simulink model "lab5_ss_decoupler"  (R2022b)
settings: Solver=VariableStepAuto  StartTime=0.0  StopTime=10.0  RelTol=1e-3
settings Model: Creator=qm-zhu  LastModifiedBy=ASUS
settings SolverCC: AlgebraicLoopSolver=TrustRegion
settings DebuggingCC: UnconnectedInputMsg=warning  UnconnectedOutputMsg=warning  UnconnectedLineMsg=warning  SFMachineParentedDataDiag=warning
settings ModelReferenceCC: EnableRefExpFcnMdlSchedulingChecks=on
settings SFSimCC: CustomCodeUndefinedFunction=UseInterfaceOnly

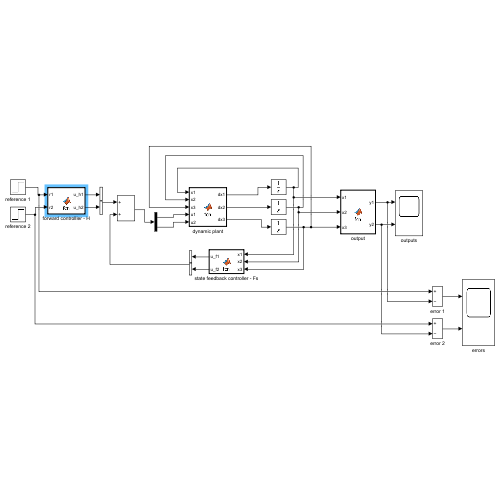
[thumbnail: Simulink's stored preview of the top-level diagram]
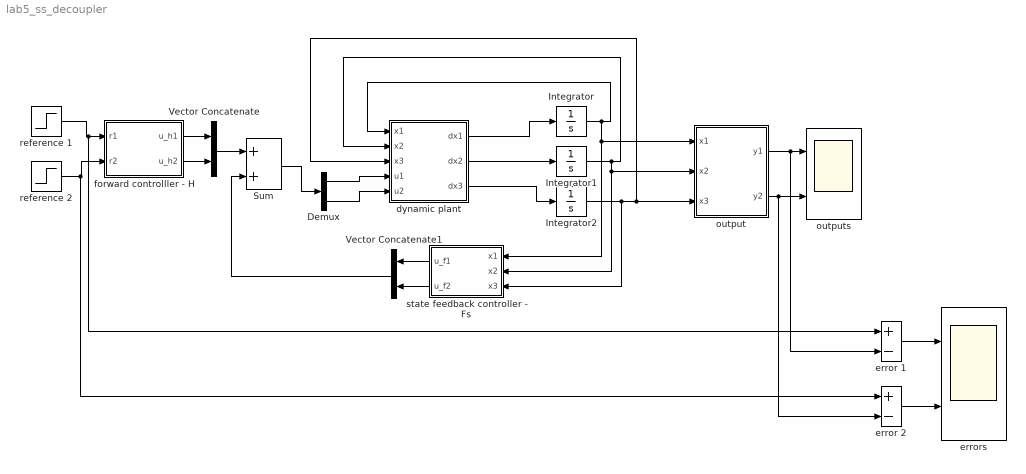
== system lab5_ss_decoupler ==
  Demux : Demux  Outputs=2
  Integrator : Integrator
  Integrator1 : Integrator
  Integrator2 : Integrator
  Sum : Sum
  Vector Concatenate : Concatenate
  Vector Concatenate1 : Concatenate
  dynamic plant : MATLAB Function  TreatAsAtomicUnit=on
  error 1 : Sum  Inputs=+-
  error 2 : Sum  Inputs=+-
  errors : Scope  NumInputPorts=2
  forward controlller - H : MATLAB Function  TreatAsAtomicUnit=on
  output : MATLAB Function  TreatAsAtomicUnit=on
  outputs : Scope  NumInputPorts=2
  reference 1 : Step  SampleTime=0
  reference 2 : Step  SampleTime=0
  state feedback controller - Fs : MATLAB Function  TreatAsAtomicUnit=on
  wires:
  dynamic plant/1(dx1) -> Integrator/1
  dynamic plant/2(dx2) -> Integrator1/1
  dynamic plant/3(dx3) -> Integrator2/1
  Integrator/1 -> state feedback controller - Fs/1(x1), output/1(x1), dynamic plant/1(x1)
  Integrator1/1 -> state feedback controller - Fs/2(x2), output/2(x2), dynamic plant/2(x2)
  Integrator2/1 -> state feedback controller - Fs/3(x3), dynamic plant/3(x3), output/3(x3)
  output/1(y1) -> error 1/2, outputs/1
  output/2(y2) -> error 2/2, outputs/2
  reference 1/1 -> error 1/1, forward controlller - H/1(r1)
  reference 2/1 -> error 2/1, forward controlller - H/2(r2)
  forward controlller - H/1(u_h1) -> Vector Concatenate/1
  forward controlller - H/2(u_h2) -> Vector Concatenate/2
  state feedback controller - Fs/1(u_f1) -> Vector Concatenate1/1
  state feedback controller - Fs/2(u_f2) -> Vector Concatenate1/2
  Vector Concatenate1/1 -> Sum/2
  Vector Concatenate/1 -> Sum/1
  Sum/1 -> Demux/1
  Demux/1 -> dynamic plant/4(u1)
  Demux/2 -> dynamic plant/5(u2)
  error 2/1 -> errors/2
  error 1/1 -> errors/1

== matlab function lab5_ss_decoupler/state feedback controller - Fs ==
  data: x1 input; u_f1 output; x2 input; x3 input; u_f2 output
function [u_f1,u_f2] = fcn(x1,x2,x3)
F_s=[-1,0,2.5;-1,-1,-2.5];
X=[x1,x2,x3]';
u_f = F_s*X;
u_f1=u_f(1,1);
u_f2=u_f(2,1);

== matlab function lab5_ss_decoupler/dynamic plant ==
  data: x1 input; x2 input; x3 input; u1 input; dx1 output; u2 input; dx2 output; dx3 output
function [dx1,dx2,dx3] = fcn(x1,x2,x3,u1,u2)
X=[x1,x2,x3]';
U=[u1,u2]';
A=[1,1,0;0,-2,0;0,1,3];
B=[1,1;-1,1;-1,1];
dx=A*X+B*U;
dx1=dx(1,1);
dx2=dx(2,1);
dx3 = dx(3,1);

== matlab function lab5_ss_decoupler/output ==
  data: x1 input; y1 output; x2 input; x3 input; y2 output
function [y1,y2] = fcn(x1,x2,x3)
X=[x1,x2,x3]';
C=[1,0,0;0,0,1];
Y=C*X;
y1=Y(1,1);
y2=Y(2,1);

== matlab function lab5_ss_decoupler/forward controlller - H ==
  data: r1 input; u_h1 output; r2 input; u_h2 output
function [u_h1,u_h2] = fcn(r1,r2)
H=[1/2,-2/2;1/2,2/2];
R=[r1,r2];
u_h=H*R';
u_h1=u_h(1,1);
u_h2=u_h(2,1);
